simulink model "test_1ph_3w_transformer"  (R2018b)
settings: Solver=FixedStepDiscrete  StartTime=0.0  StopTime=1  RelTol=1e-3
undefined symbols (not defined in the file): S2
libraries: powerlib x6, typhoonHILlib x3
settings Model: Creator=USER  LastModifiedBy=USER

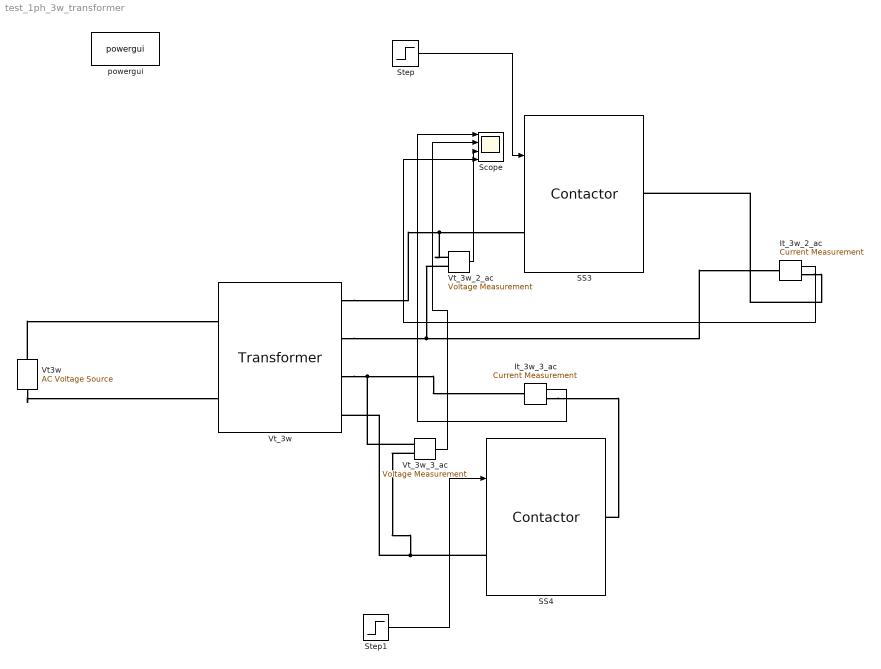
== system test_1ph_3w_transformer ==
  It_3w_2_ac : powerlib/Measurements/Current Measurement  PhasorSimulation=off  OutputType=Complex  PSBequivalent=0
  It_3w_3_ac : powerlib/Measurements/Current Measurement  PhasorSimulation=off  OutputType=Complex  PSBequivalent=0
  SS3 : typhoonHILlib/Contactor  ContType=Single Pole Single Throw  init_state=Off / S2  s1_logic=Active-high  di_1=1  tr1_delay=0  tr2_delay=0  r_on=0.001  v_f=0  r_s=1e4  c_s=inf  s0=0  toggle_init=on  old_pat=typhoonPatterns/SPST Contactor  old_size=140,184  model_loaded=off
      settings: SourceProductName=Typhoon HIL
  SS4 : typhoonHILlib/Contactor  ContType=Single Pole Single Throw  init_state=Off / S2  s1_logic=Active-high  di_1=1  tr1_delay=0  tr2_delay=0  r_on=0.001  v_f=0  r_s=1e4  c_s=inf  s0=0  toggle_init=on  old_pat=typhoonPatterns/SPST Contactor  old_size=140,184  model_loaded=off
      settings: SourceProductName=Typhoon HIL
  Scope : Scope  NumInputPorts=4
  Step : Step  Time=0.01  SampleTime=0
  Step1 : Step  Time=0.01  SampleTime=0
  Vt3w : powerlib/Electrical Sources/AC Voltage Source  Amplitude=155.5614913  Phase=0  Frequency=50  SampleTime=0  Measurements=None  BusType=swing  Pref=10e3  Qref=0  Qmin=-inf  Qmax=+inf
  Vt_3w : typhoonHILlib/Transformer  TransfType=Single-Phase Three Windings  Sn=10000  fn=50  Rm=10e3  Lm=0.5  sat_toggle=off  flux_vec=[0, 0.001, 0.005]  i_vec=[0, 1, 2]  n1=1  n2=1  coup12=off  coup13=off  coup14=off  units=SI  conn_1=Wye  V1=110  R1=0.001  L1=0.0001  I1=0  conn_2=Wye  V2=220  R2=0.004  L2=0.0004  I2=0  conn_3=Wye  V3=330  R3=0.009  L3=0.0009  I3=0  conn_4=Wye  V4=100  R4=0.1  L4=1e-3  I4=0  toggle_init=on  old_pat=typhoonPatterns/SP 3W Transformer  old_size=145,177  model_loaded=off
      settings: SourceProductName=Typhoon HIL
  Vt_3w_2_ac : powerlib/Measurements/Voltage Measurement  PhasorSimulation=off  OutputType=Complex  PSBequivalent=0
  Vt_3w_3_ac : powerlib/Measurements/Voltage Measurement  PhasorSimulation=off  OutputType=Complex  PSBequivalent=0
  powergui : powerlib/powergui  Priority=1  SimulationMode=Discrete  SampleTime=1e-6  frequency=60  Iterations=50  frequencyindice=50  Pbase=100e6  ErrMax=1e-4  UnitsV=kV  UnitsW=MW  buscounter=0  FunctionMessages=off  echomessages=off  EnableUseOfTLC=off  CurrentSourceSwitches=off  DisableSnubberDevices=off  DisableRonSwitches=off  DisableVfSwitches=off  DisplayEquations=off  SolverType=Tustin/Backward Euler (TBE)  Interpol=off  ExternalGateDelay=off  methode=off  Ts=100  x0status=blocks  SPID=on  SwTol=0  HookPort=off  RestoreLinks=warning  ResistiveCurrentMeasurement=off  Frange=[0:2:500]  Ylog=off  Xlog=on  ShowGrid=off  save=off  variable=ZData  structure=0  ZoomFFT=off  StartTime=0.0  cycles=1  DisplayStyle=1  fundamental=60  FreqAxis=off  MaxFrequency=1000  frequencyindicesteady=1  RmsSteady=1  display=off
  wires:
  Vt_3w_2_ac/1 -> Scope/3
  Vt_3w_3_ac/1 -> Scope/2
  It_3w_3_ac/1 -> Scope/1
  It_3w_2_ac/1 -> Scope/4
  Step/1 -> SS3/1
  Step1/1 -> SS4/1
  connections:
  Vt3w/RConn1 -- Vt_3w/LConn1
  Vt3w/LConn1 -- Vt_3w/LConn2
  Vt_3w/RConn1 -- Vt_3w_2_ac/LConn1 -- SS3/LConn1
  Vt_3w/RConn2 -- It_3w_2_ac/LConn1 -- Vt_3w_2_ac/LConn2
  It_3w_2_ac/RConn1 -- SS3/RConn1
  Vt_3w/RConn3 -- It_3w_3_ac/LConn1 -- Vt_3w_3_ac/LConn1
  It_3w_3_ac/RConn1 -- SS4/RConn1
  SS4/LConn1 -- Vt_3w_3_ac/LConn2 -- Vt_3w/RConn4
